simulink model "LinearVehiclePlusHaptic"  (R2018a)
settings: Solver=VariableStepAuto  StartTime=0.0  StopTime=10.0  RelTol=1e-3
values from neighbouring files (symbols this model uses):
  b = 200    [parameters_template.m]
  Ksa = 100    [LinearVehicleGains.m]
  L = 1.6    [LinearVehicleGains.m]
  R = 1/5    (= 0.2)    [LinearVehicleGains.m]    (also in parameters_template.m)
  tau = 0.0001    [LinearVehicleGains.m]
undefined symbols (not defined in the file or in its folder): J, k, Kd, Kdm, Kp, Kpm
settings Model: Creator=salman  LastModifiedBy=ddhanush

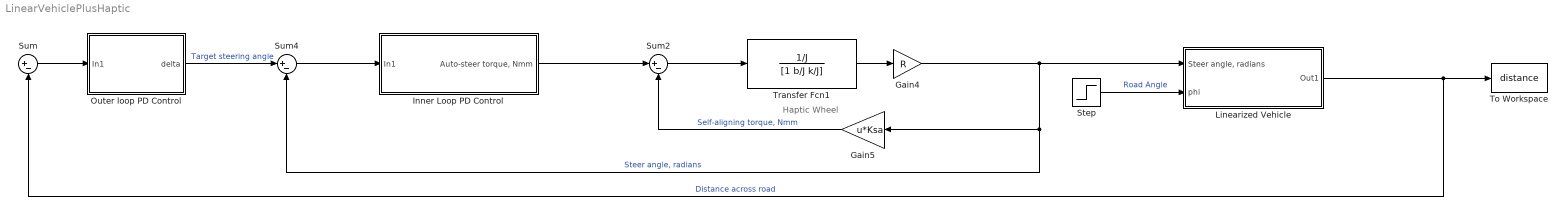
== system LinearVehiclePlusHaptic ==
  note: Haptic Wheel
  Gain4 : Gain  Gain=R
  Gain5 : Gain  Gain=u*Ksa
  Inner Loop PD Control : Subsystem
  Linearized Vehicle : Subsystem
  Outer loop PD Control : Subsystem
  Step : Step  SampleTime=0
  Sum : Sum  Inputs=|+-
  Sum2 : Sum  Inputs=|+-
  Sum4 : Sum  Inputs=|+-
  To Workspace : ToWorkspace  VariableName=distance  SampleTime=-1
  Transfer Fcn1 : TransferFcn  Numerator=1/J  Denominator=[1 b/J k/J]
  wires:
  Gain5/1 -> Sum2/2  "Self-aligning torque, Nmm"
  Outer loop PD Control/1(delta) -> Sum4/1  "Target steering angle"
  Sum2/1 -> Transfer Fcn1/1
  Transfer Fcn1/1 -> Gain4/1
  Gain4/1 -> Linearized Vehicle/1("Steer angle, radians"), Gain5/1, Sum4/2  "Steer angle, radians"
  Sum4/1 -> Inner Loop PD Control/1(In1)
  Inner Loop PD Control/1("Auto-steer torque, Nmm") -> Sum2/1
  Linearized Vehicle/1(Out1) -> To Workspace/1, Sum/2  "Distance across road"
  Sum/1 -> Outer loop PD Control/1(In1)
  ? -> Sum/1  "n_desired"
  Step/1 -> Linearized Vehicle/2(phi)  "Road Angle"

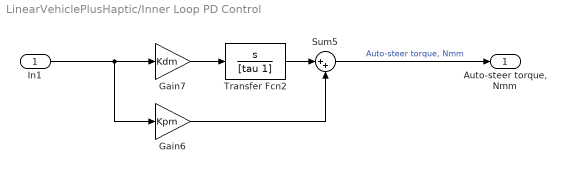
== system LinearVehiclePlusHaptic/Inner Loop PD Control ==
  In1 : Inport
  Gain6 : Gain  Gain=Kpm
  Gain7 : Gain  Gain=Kdm
  Sum5 : Sum  Inputs=|++
  Transfer Fcn2 : TransferFcn  Numerator=[1 0]  Denominator=[tau 1]
  "Auto-steer torque, Nmm" : Outport
  wires:
  Gain7/1 -> Transfer Fcn2/1
  Sum5/1 -> "Auto-steer torque, Nmm"/1  "Auto-steer torque, Nmm"
  Gain6/1 -> Sum5/2
  In1/1 -> Gain6/1, Gain7/1
  Transfer Fcn2/1 -> Sum5/1

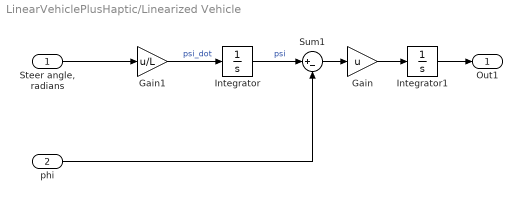
== system LinearVehiclePlusHaptic/Linearized Vehicle ==
  "Steer angle, radians" : Inport
  phi : Inport  Port=2
  Gain : Gain  Gain=u
  Gain1 : Gain  Gain=u/L
  Integrator : Integrator
  Integrator1 : Integrator
  Sum1 : Sum  Inputs=|+-
  Out1 : Outport
  wires:
  phi/1 -> Sum1/2
  Gain/1 -> Integrator1/1
  Gain1/1 -> Integrator/1  "psi_dot"
  Integrator1/1 -> Out1/1
  Integrator/1 -> Sum1/1  "psi"
  "Steer angle, radians"/1 -> Gain1/1
  Sum1/1 -> Gain/1

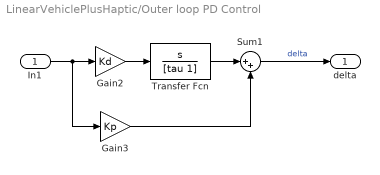
== system LinearVehiclePlusHaptic/Outer loop PD Control ==
  In1 : Inport
  Gain2 : Gain  Gain=Kd
  Gain3 : Gain  Gain=Kp
  Sum1 : Sum  Inputs=|++
  Transfer Fcn : TransferFcn  Numerator=[1 0]  Denominator=[tau 1]
  delta : Outport
  wires:
  Sum1/1 -> delta/1  "delta"
  Gain3/1 -> Sum1/2
  In1/1 -> Gain3/1, Gain2/1
  Gain2/1 -> Transfer Fcn/1
  Transfer Fcn/1 -> Sum1/1
